simulink model "hw1code"  (R2022b)
settings: Solver=VariableStepAuto  StartTime=0.0  StopTime=10.0  RelTol=1e-3
undefined symbols (not defined in the file): Va
settings Model: Creator=junseo  LastModifiedBy=junseo

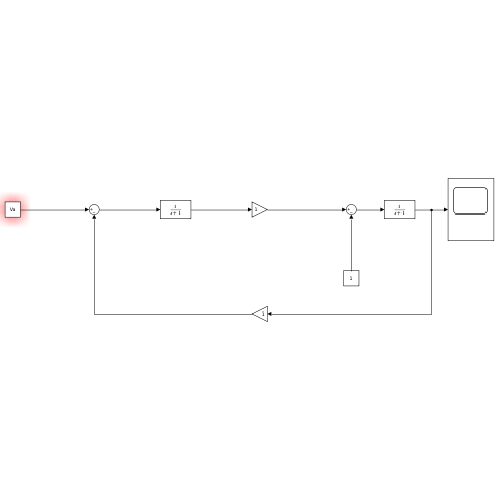
[thumbnail: Simulink's stored preview of the top-level diagram]
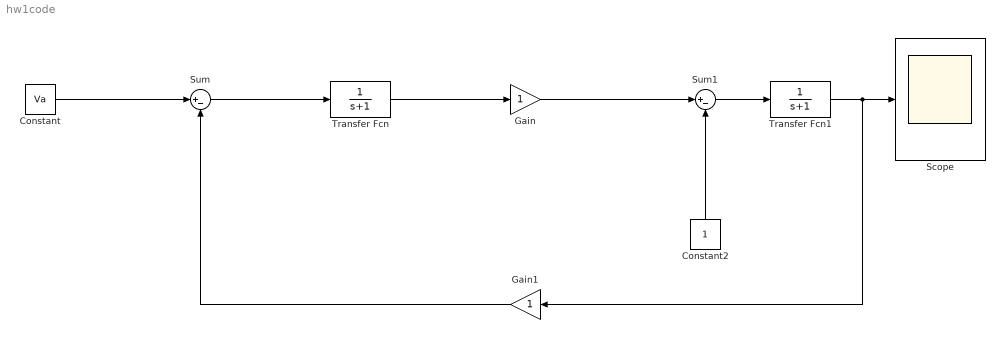
== system hw1code ==
  Constant : Constant  Value=Va  VectorParams1D=off
  Constant2 : Constant
  Gain : Gain
  Gain1 : Gain
  Scope : Scope
  Sum : Sum  Inputs=|+-
  Sum1 : Sum  Inputs=|+-
  Transfer Fcn : TransferFcn  Denominator=[1 1]
  Transfer Fcn1 : TransferFcn  Denominator=[1 1]
  wires:
  Gain/1 -> Sum1/1
  Constant2/1 -> Sum1/2
  Sum1/1 -> Transfer Fcn1/1
  Transfer Fcn1/1 -> Gain1/1, Scope/1
  Constant/1 -> Sum/1
  Gain1/1 -> Sum/2
  Sum/1 -> Transfer Fcn/1
  Transfer Fcn/1 -> Gain/1
